simulink model "ModelCTClean"  (R2020b)
settings: Solver=VariableStepAuto  StartTime=0.0  StopTime=7  RelTol=1e-3
values from neighbouring files (symbols this model uses):
  Power = [0 0.135039524161 8.91914965689 7.78138466797 9.0073673393 8.96604203154 8.86759000228 15.68308669 17.9316117445 18.8693109472 25.7680840998 34.2690025221 ... (50 elements, 50x1)]    [MotorData.mat]    (also in OptimisationData.mat = [0 0.134792669981 8.9180951627 7.77881648635 9.00749423422 8)
  Throttle = [0 1 2.66666666667 3.44444444444 6.55555555556 8.11111111111 8.88888888889 13.6666666667 14.4444444444 15.2222222222 18.3333333333 21.5555555556 ... (50 elements, 50x1)]    [MotorData.mat]    (also in OptimisationData.mat)
  Thrust = [0 0.00386703849483 0.447248955951 0.381725752671 0.429816366755 0.448130327307 0.434268732353 0.786362880096 0.850043356053 0.907127881895 1.24377109743 1.5194958901 ... (50 elements, 50x1)]    [MotorData.mat]    (also in OptimisationData.mat)
libraries: simulink x1
settings Model: Creator=IR13  LastModifiedBy=IR13
settings SolverCC: ZeroCrossAlgorithm=Adaptive
settings DebuggingCC: IgnoredZcDiagnostic=none

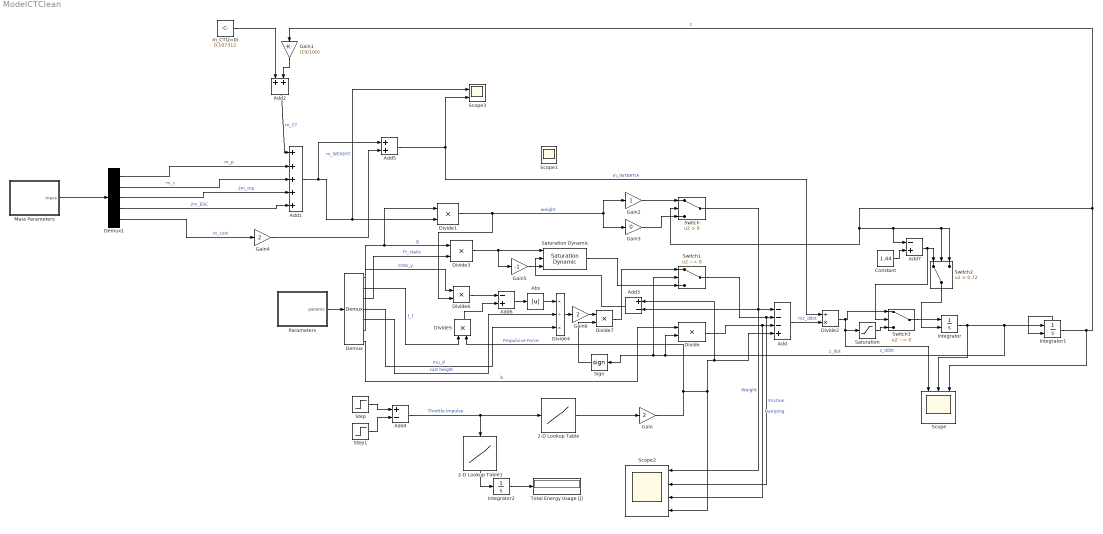
== system ModelCTClean ==
  2-D Lookup Table : Lookup_n-D  NumberOfTableDimensions=1  BreakpointsForDimension1=Throttle  BreakpointsForDimension2=[1:3]  Table=Thrust  InterpMethod=Cubic spline  ExtrapMethod=Clip  InternalRulePriority=Speed  RndMeth=Simplest  InputSameDT=on
  2-D Lookup Table1 : Lookup_n-D  NumberOfTableDimensions=1  BreakpointsForDimension1=Throttle  BreakpointsForDimension2=[1:3]  Table=Power  InterpMethod=Cubic spline  ExtrapMethod=Clip  InternalRulePriority=Speed  RndMeth=Simplest  InputSameDT=on
  Abs : Abs
  Add : Sum  Inputs=---+
  Add1 : Sum  Inputs=+++++
  Add2 : Sum
  Add3 : Sum  Inputs=+-
  Add4 : Sum  Inputs=+-
  Add5 : Sum
  Add6 : Sum  Inputs=-+
  Add7 : Sum  Inputs=-+
  Constant : Constant  Value=1.44
  Demux : Demux  Outputs=7
  Demux1 : Demux  Outputs=5
  Divide{,1,3,5..7} (6 alike) : Product  Inputs=**
  Divide2 : Product  Inputs=/*
  Divide4 : Product  Inputs=*/*
  Gain : Gain  Gain=2
  Gain1 : Gain  Gain=(19/100)
  Gain2 : Gain
  Gain3 : Gain  Gain=0
  Gain4 : Gain  Gain=2
  Gain5 : Gain  Gain=-1
  Gain6 : Gain  Gain=2
  Integrator : Integrator  ExternalReset=falling
  Integrator1 : Integrator  ExternalReset=falling  ShowStatePort=on
  Integrator2 : Integrator
  Mass Parameters : MATLAB Function  TreatAsAtomicUnit=on
  Parameters : MATLAB Function  TreatAsAtomicUnit=on
  Saturation : Saturate  UpperLimit=0  LowerLimit=-inf
  Saturation Dynamic : simulink/Discontinuities/Saturation Dynamic  OutMin=[]  OutMax=[]  OutDataTypeStr=Inherit: Same as second input  OutDataType=fixdt(1, 16)  OutScaling=2^-10  DoSatur=off
  Scope : Scope  NumInputPorts=3
  Scope2 : Scope  NumInputPorts=4
  Scope3 : Scope  NumInputPorts=2
  Sign : Signum
  Step : Step  Time=2  After=100  SampleTime=0
  Step1 : Step  Time=3  After=100  SampleTime=0
  Switch : Switch  Criteria=u2 > Threshold
  Switch1 : Switch  Criteria=u2 ~= 0
  Switch2 : Switch  Criteria=u2 > Threshold  Threshold=0.72
  Switch3 : Switch  Criteria=u2 ~= 0
  Total Energy Usage [J] : Display
  m_CT(z=0) : Constant  Value=0.107312
  Scope1 : Scope
  wires:
  Divide1/1 -> Divide6/2, Gain3/1, Gain2/1  "weight"
  Integrator/1 -> Scope/2, Integrator1/1, Sign/1, Switch1/2, Divide/2  "z_dot"
  Demux/7 -> Divide/1  "b"
  Step/1 -> Add4/1
  Add3/1 -> Saturation Dynamic/2
  Step1/1 -> Add4/2
  Add/1 -> Divide2/2  "mz_ddot"
  Integrator1/State -> Integrator1/2
  Gain2/1 -> Switch/1
  Gain3/1 -> Switch/3
  Saturation Dynamic/1 -> Switch1/3
  Add4/1 -> 2-D Lookup Table1/1, 2-D Lookup Table/1  "Throttle Impulse"
  Parameters/1(params) -> Demux/1
  Demux/1 -> Divide1/1, Divide3/1  "g"
  Demux/3 -> Divide3/2  "Fr_static"
  Divide3/1 -> Gain5/1, Saturation Dynamic/1
  Gain5/1 -> Saturation Dynamic/3
  Demux/4 -> Divide4/3  "mu_d"
  Demux/5 -> Divide4/2  "cart height"
  Demux/6 -> Divide6/1  "COG_y"
  Divide4/1 -> Gain6/1
  Gain/1 -> Scope2/4, Add/4, Add3/1, Divide5/2  "Propulsive Force"
  Divide/1 -> Add/3, Scope2/3  "Damping"
  Switch1/1 -> Add/2, Scope2/2  "Friction"
  Switch/1 -> Scope2/1, Add3/2, Add/1  "Weight"
  Integrator1/1 -> Scope/3, Gain1/1, Add7/1, Switch2/3, Switch2/2, Switch/2  "z"
  Add1/1 -> Add5/1, Scope3/1, Divide1/2  "m_WEIGHT"
  Add5/1 -> Scope3/2, Divide2/1  "m_INTERTIA"
  Demux1/1 -> Add1/2  "m_p"
  Demux1/2 -> Add1/3  "m_s"
  Demux1/3 -> Add1/4  "2m_mp"
  Demux1/4 -> Add1/5  "2m_ESC"
  Demux1/5 -> Gain4/1  "m_cart"
  m_CT(z=0)/1 -> Add2/1
  Gain1/1 -> Add2/2
  Add2/1 -> Add1/1  "m_CT"
  Gain4/1 -> Add5/2
  Mass Parameters/1(mass) -> Demux1/1
  Demux/2 -> Divide5/1  "l_T"
  2-D Lookup Table/1 -> Gain/1
  2-D Lookup Table1/1 -> Integrator2/1
  Integrator2/1 -> Total Energy Usage [J]/1
  Divide5/1 -> Add6/2
  Divide6/1 -> Add6/1
  Add6/1 -> Abs/1
  Abs/1 -> Divide4/1
  Switch2/1 -> Integrator/2
  Add7/1 -> Switch2/1, Switch3/2
  Constant/1 -> Add7/2
  Divide2/1 -> Scope/1, Saturation/1, Switch3/1  "z_ddot"
  Switch3/1 -> Integrator/1
  Saturation/1 -> Switch3/3
  Gain6/1 -> Divide7/1
  Divide7/1 -> Switch1/1
  Sign/1 -> Divide7/2

== matlab function ModelCTClean/Parameters ==
  data: params output
function params = fcn()

%raw parameters
g = 9.81;
lT = 10; %y position of thrust point [mm]
F_r_static = 0.13; %static friction force [kgf]
mu_d = 0.14; %dynamic friction coefficient 
cart_height = 210.4; %[mm]
CoG_y = 10; %%[mm]
b = 0.2; %damping constant

params = [g;lT;F_r_static; mu_d; cart_height;CoG_y;b];

== matlab function ModelCTClean/Mass Parameters ==
  data: mass output
function mass = fcn()

%raw parameters

m_p = 0.15;
m_s = 0.2;
m_mp = 0.202; %mass of one motor prop
m_ESC = 0.102;
m_cart = 0.4; %mass of one cart without additional stuff


mass = [m_p;m_s;m_mp;m_ESC;m_cart];
